simulink model "penduloDobleEnsambleconfunciones"  (R2013a)
settings: Solver=ode45  StartTime=0.0  StopTime=inf  RelTol=1e-3
values from neighbouring files (symbols this model uses):
  g = 9.81    [Parametros_Pendulo_Doble.m]
  Theta1 = (m1*lc1^2)+(m2*l1^2)+I1    (= 0.09775488)    [Parametros_Pendulo_Doble.m]
  Theta2 = (m2*lc2^2)+I2    (= 0.00775807)    [Parametros_Pendulo_Doble.m]
  Theta3 = (m2*l1*lc2)    (= 0.008897)    [Parametros_Pendulo_Doble.m]
  Theta4 = (m1*lc1)+(m2*l1)    (= 0.495148)    [Parametros_Pendulo_Doble.m]
  Theta5 = (m2*lc2)    (= 0.044485)    [Parametros_Pendulo_Doble.m]
undefined symbols (not defined in the file or in its folder): perno
libraries: mblibv1 x16
settings Model: Creator=LornBaltymor  LastModifiedBy=Daniel
settings SimMechanicsCC: VisOnUpdateDiagram=on  VisDuringSimulation=on

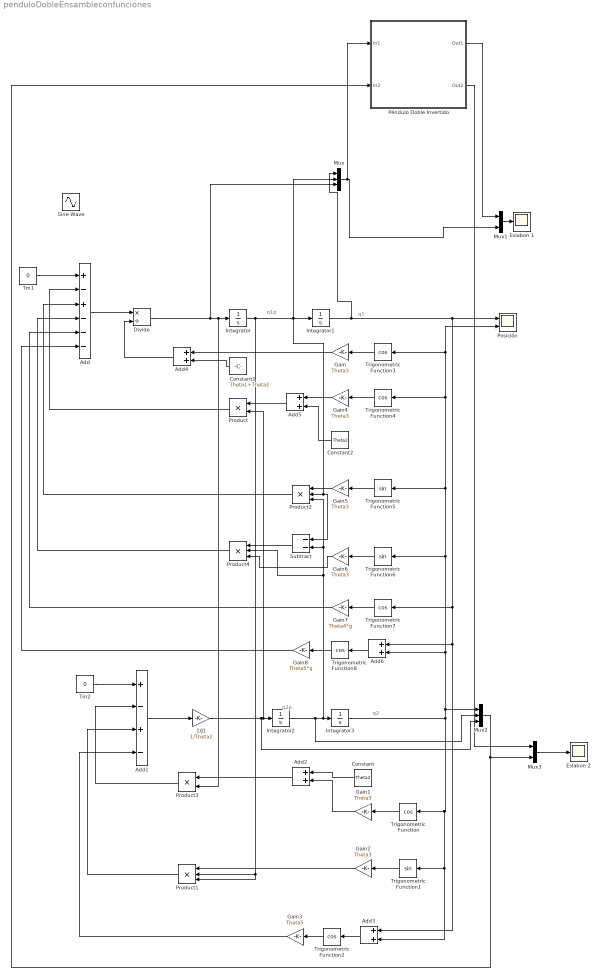
== system penduloDobleEnsambleconfunciones ==
  note: q2
  note: q1
  note: q1p
  note: q2p
  1/J1 : Gain  Gain=1/Theta2
  Add : Sum  Inputs=+-+---
  Add1 : Sum  Inputs=+-+-
  Add{2..6} (5 alike) : Sum
  Constant : Constant  Value=Theta2
  Constant1 : Constant  Value=Theta1+Theta2
  Constant2 : Constant  Value=Theta2
  Divide : Product  Inputs=*/
  Eslabon 1 : Scope
      settings: YMin=-1000  YMax=12000
  "Eslabon 2 " : Scope
      settings: YMin=-1000  YMax=12000  SaveName=ScopeData2
  Gain{,1..2,4..6} (6 alike) : Gain  Gain=Theta3
  Gain3 : Gain  Gain=Theta5
  Gain7 : Gain  Gain=Theta4*g
  Gain8 : Gain  Gain=Theta5*g
  Integrator : Integrator
  Integrator1 : Integrator  InitialCondition=pi/2
  Integrator2 : Integrator
  Integrator3 : Integrator  InitialCondition=pi/2
  Mux : Mux  Inputs=3
  Mux1 : Mux  Inputs=2
  Mux2 : Mux  Inputs=3
  Mux3 : Mux  Inputs=2
  Posición : Scope  NumInputPorts=2
      settings: YMin=86700~-3.21  YMax=88100~-3.07
  Product : Product
  Product1 : Product  Inputs=3
  Product2 : Product  Inputs=3
  Product3 : Product
  Product4 : Product  Inputs=3
  Péndulo Doble Invertido : Subsystem
  Sine Wave : Sin  SampleTime=0
  Subtract : Sum  Inputs=--
  Tm1 : Constant  Value=0
  Tm2 : Constant  Value=0
  Trigonometric Function{,2..4,7..8} (6 alike) : Trigonometry  Operator=cos
  Trigonometric Function1 : Trigonometry
  Trigonometric Function5 : Trigonometry
  Trigonometric Function6 : Trigonometry
  wires:
  Tm2/1 -> Add1/1
  Add1/1 -> 1/J1/1
  1/J1/1 -> Mux2/3, Product/2, Integrator2/1
  Integrator1/1 -> Mux/1, Trigonometric Function7/1, Add6/1, Add3/1, Posición/1
  Integrator2/1 -> Mux2/2, Product4/2, Subtract/2, Product2/3, Integrator3/1
  Divide/1 -> Mux/3, Product3/2, Integrator/1
  Integrator/1 -> Subtract/1, Product2/2, Mux/2, Integrator1/1, Product1/3, Product1/2
  Product3/1 -> Add1/2
  Constant/1 -> Add2/1
  Gain1/1 -> Add2/2
  Trigonometric Function/1 -> Gain1/1
  Integrator3/1 -> Mux2/1, Add6/2, Trigonometric Function6/1, Trigonometric Function5/1, Trigonometric Function4/1, Trigonometric Function3/1, Posición/2, Add3/2, Trigonometric Function1/1, Trigonometric Function/1
  Add2/1 -> Product3/1
  Trigonometric Function1/1 -> Gain2/1
  Gain2/1 -> Product1/1
  Product1/1 -> Add1/3
  Trigonometric Function2/1 -> Gain3/1
  Gain3/1 -> Add1/4
  Add3/1 -> Trigonometric Function2/1
  Trigonometric Function3/1 -> Gain/1
  Gain/1 -> Add4/1
  Constant1/1 -> Add4/2
  Add4/1 -> Divide/2
  Add/1 -> Divide/1
  Trigonometric Function4/1 -> Gain4/1
  Gain4/1 -> Add5/1
  Constant2/1 -> Add5/2
  Add5/1 -> Product/1
  Product/1 -> Add/2
  Trigonometric Function5/1 -> Gain5/1
  Gain5/1 -> Product2/1
  Product2/1 -> Add/3
  Subtract/1 -> Product4/1
  Gain6/1 -> Product4/3
  Trigonometric Function6/1 -> Gain6/1
  Product4/1 -> Add/4
  Trigonometric Function7/1 -> Gain7/1
  Gain7/1 -> Add/5
  Trigonometric Function8/1 -> Gain8/1
  Add6/1 -> Trigonometric Function8/1
  Gain8/1 -> Add/6
  Mux/1 -> Péndulo Doble Invertido/1(In1), Mux1/2
  Mux1/1 -> Eslabon 1/1
  Péndulo Doble Invertido/1(Out1) -> Mux1/1
  Mux2/1 -> Mux3/2, Péndulo Doble Invertido/2(In2)
  Péndulo Doble Invertido/2(Out2) -> Mux3/1
  Mux3/1 -> "Eslabon 2 "/1
  Tm1/1 -> Add/1

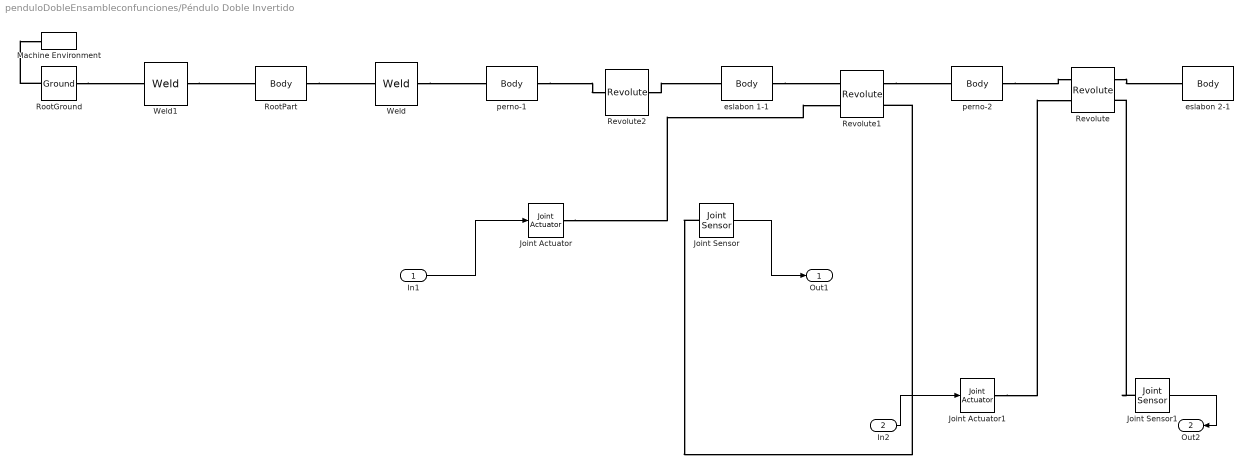
== system penduloDobleEnsambleconfunciones/Péndulo Doble Invertido ==
  In1 : Inport
  In2 : Inport  Port=2
  Joint Actuator : mblibv1/Sensors &  Actuators/Joint Actuator  UpdateFromCAD=off  PhysicalDomain=Mechanical  PortType=blob  ActuationStyle=Motion  AngleUnits=deg  ArcVelocityUnits=deg/s  ArcAccelerationUnits=deg/s^2  CoordPositionUnits=m  VelocityUnits=m/s  AccelerationUnits=m/s^2  ForceUnits=N  TorqueUnits=N*m  ActiveIO=on  Width=3  DialogClass=MechanicalActuatorBlock  Primitive=R1  ReferenceFrame=Absolute (World)
  Joint Actuator1 : mblibv1/Sensors &  Actuators/Joint Actuator  UpdateFromCAD=off  PhysicalDomain=Mechanical  PortType=blob  ActuationStyle=Motion  AngleUnits=deg  ArcVelocityUnits=deg/s  ArcAccelerationUnits=deg/s^2  CoordPositionUnits=m  VelocityUnits=m/s  AccelerationUnits=m/s^2  ForceUnits=N  TorqueUnits=N*m  ActiveIO=on  Width=3  DialogClass=MechanicalActuatorBlock  Primitive=R1  ReferenceFrame=Absolute (World)
  Joint Sensor : mblibv1/Sensors &  Actuators/Joint Sensor  UpdateFromCAD=off  PhysicalDomain=Mechanical  PortType=blob  Muxed=on  Pose=off  Angle=on  AngleUnits=deg  ArcVelocity=off  ArcVelocityUnits=deg/s  ArcAcceleration=off  ArcAccelerationUnits=deg/s^2  CoordPosition=on  CoordPositionUnits=m  Velocity=off  VelocityUnits=m/s  Acceleration=off  AccelerationUnits=m/s^2  Quaternion=on  QuaternionDT=off  QuaternionDDT=off  QuaternionUnits=off  OutputVector=[1]  ActiveIO=on  Width=1  DialogClass=MechanicalSensorBlock  Primitive=R1  Force=off  ForceUnits=N  Torque=off  TorqueUnits=N*m  ReferenceFrame=Absolute (World)  ReactionSensedSide=Base  ReactionReferenceFrame=Absolute (World)  ReactionForce=off  ReactionForceUnits=N  ReactionMoment=off  ReactionMomentUnits=N*m
  Joint Sensor1 : mblibv1/Sensors &  Actuators/Joint Sensor  UpdateFromCAD=off  PhysicalDomain=Mechanical  PortType=blob  Muxed=on  Pose=off  Angle=on  AngleUnits=deg  ArcVelocity=off  ArcVelocityUnits=deg/s  ArcAcceleration=off  ArcAccelerationUnits=deg/s^2  CoordPosition=on  CoordPositionUnits=m  Velocity=off  VelocityUnits=m/s  Acceleration=off  AccelerationUnits=m/s^2  Quaternion=on  QuaternionDT=off  QuaternionDDT=off  QuaternionUnits=off  OutputVector=[1]  ActiveIO=on  Width=1  DialogClass=MechanicalSensorBlock  Primitive=R1  Force=off  ForceUnits=N  Torque=off  TorqueUnits=N*m  ReferenceFrame=Absolute (World)  ReactionSensedSide=Base  ReactionReferenceFrame=Absolute (World)  ReactionForce=off  ReactionForceUnits=N  ReactionMoment=off  ReactionMomentUnits=N*m
  Machine Environment : mblibv1/Bodies/Machine Environment  PortType=env  PhysicalDomain=Mechanical  DialogTemplateClass=MECH.MachineEnvironment  SyncWhenCopied=off  Gravity=[0 -9.81 0]  GravityUnits=m/s^2  GravityAsSignal=off  Dimensionality=Auto-detect  AnalysisType=Forward dynamics  LinearAssemblyTolerance=1e-3  LinearAssemblyToleranceUnits=m  AngularAssemblyTolerance=1e-3  AngularAssemblyToleranceUnits=rad  ConstraintSolverType=Stabilizing  ConstraintRelTolerance=1e-4  ConstraintAbsTolerance=1e-4  UseRobustSingularityHandling=off  RedundancyAnalysisToleranceType=Automatically select tolerance  RedundancyAnalysisTolerance=1e-14  StatePerturbationType=Fixed  PerturbationSize=1e-5  VisualizeMachine=on  BodyVisualizationType=Use model default body geometries  BodyColorSelMode=Use model default  DefaultBodyColor=[1 0 0]
  Revolute : mblibv1/Joints/Revolute  LConnTagsString=__newl0|SA1  RConnTagsString=__newr0|SA1  UpdateFromCAD=on  PMImportedID=eslabon 2-1:-:perno-2  NumSAPorts=2  CutJoint=off  MarkAsCut=off  Primitives=prismatic  PrimitiveProps=R1$World$[0,0,-1]$revolute  DialogClass=JointBlock  R1Axis=[0,0,-1]
  Revolute1 : mblibv1/Joints/Revolute  LConnTagsString=__newl0|SA1  RConnTagsString=__newr0|SA1  UpdateFromCAD=on  PMImportedID=eslabon 1-1:-:perno-2  NumSAPorts=2  CutJoint=off  MarkAsCut=off  Primitives=prismatic  PrimitiveProps=R1$World$[0,0,1]$revolute  DialogClass=JointBlock  R1Axis=[0,0,1]
  Revolute2 : mblibv1/Joints/Revolute  LConnTagsString=__newl0  RConnTagsString=__newr0  UpdateFromCAD=on  PMImportedID=eslabon 1-1:-:perno-1  NumSAPorts=0  CutJoint=off  MarkAsCut=off  Primitives=prismatic  PrimitiveProps=R1$World$[0,0,1]$revolute  DialogClass=JointBlock  R1Axis=[0,0,1]
  RootGround : mblibv1/Bodies/Ground  UpdateFromCAD=on  PMImportedID=RootGround  LeftPortType=env  RightPortType=workingframe  PhysicalDomain=Mechanical  DialogClass=GroundBlock  CoordPosition=[0.0411534,0.0510219,0.0512834]  CoordPositionUnits=m  StateVectorMgrId=2  MachineId=[3 0]  ShowEnvPort=on
  RootPart : mblibv1/Bodies/Body  LConnTagsString=CS3  RConnTagsString=CS2  UpdateFromCAD=on  PMImportedID=pendulo doble ensamble/RootPart  DialogClass=MechanicalBodyBlock  Mass=0  MassUnits=kg  InertiaUnits=kg*m^2  Inertia=[0,0,0;0,0,0;0,0,0]  Shape=Cylinder  ShapeDims=[1 1]  ShapeUnits=m  ShapeUse=false  Density=1  DensityUnits=kg/m^3  DensityUse=false  GraphicsMode=MACHINE_DEFAULT  BodyColorSelMode=MACHINE_DEFAULT  BodyColor=[1;0;0]  AttachedToCS=CS1  CG=Right$CG$[0.0411534 0.0510219 0.0512834]$WORLD$WORLD$m$[1 0 0;0 1 0;0 0 1]$3x3 Transform$rad$WORLD$false$pendulo doble ensamble/RootPart::CG(AUTOGEN)  WorkingFrames=Right$CS1$[0 0 0]$WORLD$WORLD$m$[1 0 0;0 1 0;0 0 1]$3x3 Transform$rad$WORLD$false$pendulo doble ensamble/RootPart::CS1(AUTOGEN)#Right$CS2$[0.000634377 -0.00147675 0.05]$WORLD$WORLD$m$[1 0 0;0 1 0;0 0 1]$3x3 Transform$rad$WORLD$true$pendulo doble ensamble/RootPart:-:perno-1::pendulo doble ensamble/RootPart(AUTOGEN)#Left$CS3$[0.0411534 0.0510219 0.0512834]$WORLD$WORLD$m$[1 0 0;0 1 0;0 0 1]$3x3 Transform$rad$WORLD$true$RootGround:-:pendulo doble ensamble/RootPart::pendulo doble ensamble/RootPart(AUTOGEN)  CGPos=[0.0411534 0.0510219 0.0512834]  CGRot=[1 0 0;0 1 0;0 0 1]  CS0Pos=[]  CS0Rot=[]  CS1Pos=[0 0 0]  CS1Rot=[1 0 0;0 1 0;0 0 1]  CS2Pos=[0.000634377 -0.00147675 0.05]  CS2Rot=[1 0 0;0 1 0;0 0 1]  CS3Pos=[0.0411534 0.0510219 0.0512834]  CS3Rot=[1 0 0;0 1 0;0 0 1]  CS4Pos=[]  CS4Rot=[]  CS5Pos=[]  CS5Rot=[]  CS6Pos=[]  CS6Rot=[]  CS7Pos=[]  CS7Rot=[]  CS8Pos=[]  CS8Rot=[]  CS9Pos=[]  CS9Rot=[]  CS10Pos=[]  CS10Rot=[]  CS11Pos=[]  CS11Rot=[]  CS12Pos=[]  CS12Rot=[]  CS13Pos=[]  CS13Rot=[]  CS14Pos=[]  CS14Rot=[]  CS15Pos=[]  CS15Rot=[]  CS16Pos=[]  CS16Rot=[]  CS17Pos=[]  CS17Rot=[]  CS18Pos=[]  CS18Rot=[]  CS19Pos=[]  CS19Rot=[]  CS20Pos=[]  CS20Rot=[]
  Weld : mblibv1/Joints/Weld  LConnTagsString=__newl0  RConnTagsString=__newr0  UpdateFromCAD=on  PMImportedID=pendulo doble ensamble/RootPart:-:perno-1  NumSAPorts=0  CutJoint=off  MarkAsCut=off  Primitives=weld  PrimitiveProps=W$WORLD$[0.57735,0.57735,0.57735]$weld  DialogClass=JointBlock  WAxis=[0.57735,0.57735,0.57735]
  Weld1 : mblibv1/Joints/Weld  LConnTagsString=__newl0  RConnTagsString=__newr0  UpdateFromCAD=on  PMImportedID=RootGround:-:pendulo doble ensamble/RootPart  NumSAPorts=0  CutJoint=off  MarkAsCut=off  Primitives=weld  PrimitiveProps=W$WORLD$[0.57735,0.57735,0.57735]$weld  DialogClass=JointBlock  WAxis=[0.57735,0.57735,0.57735]
  eslabon 1-1 : mblibv1/Bodies/Body  LConnTagsString=CS3  RConnTagsString=CS2  UpdateFromCAD=on  PMImportedID=eslabon 1-1  DialogClass=MechanicalBodyBlock  Mass=0.0368584  MassUnits=kg  InertiaUnits=kg*m^2  Inertia=[2.95158e-05,0,0;0,2.54231e-06,0;0,0,2.96008e-05]  Shape=Cylinder  ShapeDims=[1 1]  ShapeUnits=m  ShapeUse=false  Density=1  DensityUnits=kg/m^3  DensityUse=false  GraphicsMode=GFXFILE  GraphicsFileName=pendulo doble ensamble - eslabon 1-1.STL  BodyColorSelMode=COLORPALETTE  BodyColor=[0.792157;0.819608;0.933333]  AttachedToCS=CS1  CG=Right$CG$[0.0289122 0.0268139 0.065]$WORLD$WORLD$m$[-0.707267 -0.706946 0;0.706946 -0.707267 0;0 0 1]$3x3 Transform$rad$WORLD$false$eslabon 1-1::CG(AUTOGEN)  WorkingFrames=Right$CS1$[0.0642596 0.0621773 0.065]$WORLD$WORLD$m$[-0.707267 -0.706946 0;0.706946 -0.707267 0;0 0 1]$3x3 Transform$rad$WORLD$false$eslabon 1-1::CS1(AUTOGEN)#Right$CS2$[0.0571901 0.0551046 0.075]$WORLD$WORLD$m$[1 0 0;0 1 0;0 0 1]$3x3 Transform$rad$WORLD$true$eslabon 1-1:-:perno-2::eslabon 1-1(AUTOGEN)#Left$CS3$[0.000634377 -0.00147675 0.075]$WORLD$WORLD$m$[1 0 0;0 1 0;0 0 1]$3x3 Transform$rad$WORLD$true$eslabon 1-1:-:perno-1::eslabon 1-1(AUTOGEN)  CGPos=[0.0289122 0.0268139 0.065]  CGRot=[-0.707267 -0.706946 0;0.706946 -0.707267 0;0 0 1]  CS0Pos=[]  CS0Rot=[]  CS1Pos=[0.0642596 0.0621773 0.065]  CS1Rot=[-0.707267 -0.706946 0;0.706946 -0.707267 0;0 0 1]  CS2Pos=[0.0571901 0.0551046 0.075]  CS2Rot=[1 0 0;0 1 0;0 0 1]  CS3Pos=[0.000634377 -0.00147675 0.075]  CS3Rot=[1 0 0;0 1 0;0 0 1]  CS4Pos=[]  CS4Rot=[]  CS5Pos=[]  CS5Rot=[]  CS6Pos=[]  CS6Rot=[]  CS7Pos=[]  CS7Rot=[]  CS8Pos=[]  CS8Rot=[]  CS9Pos=[]  CS9Rot=[]  CS10Pos=[]  CS10Rot=[]  CS11Pos=[]  CS11Rot=[]  CS12Pos=[]  CS12Rot=[]  CS13Pos=[]  CS13Rot=[]  CS14Pos=[]  CS14Rot=[]  CS15Pos=[]  CS15Rot=[]  CS16Pos=[]  CS16Rot=[]  CS17Pos=[]  CS17Rot=[]  CS18Pos=[]  CS18Rot=[]  CS19Pos=[]  CS19Rot=[]  CS20Pos=[]  CS20Rot=[]
  eslabon 2-1 : mblibv1/Bodies/Body  LConnTagsString=CS2  UpdateFromCAD=on  PMImportedID=eslabon 2-1  DialogClass=MechanicalBodyBlock  Mass=0.0304292  MassUnits=kg  InertiaUnits=kg*m^2  Inertia=[1.65845e-05,0,0;0,2.07116e-06,0;0,0,1.6627e-05]  Shape=Cylinder  ShapeDims=[1 1]  ShapeUnits=m  ShapeUse=false  Density=1  DensityUnits=kg/m^3  DensityUse=false  GraphicsMode=GFXFILE  GraphicsFileName=pendulo doble ensamble - eslabon 2-1.STL  BodyColorSelMode=COLORPALETTE  BodyColor=[0.792157;0.819608;0.933333]  AttachedToCS=CS1  CG=Right$CG$[0.0591404 0.0865929 0.035]$WORLD$WORLD$m$[-0.998087 -0.0618188 0;0.0618188 -0.998087 0;0 0 1]$3x3 Transform$rad$WORLD$false$eslabon 2-1::CG(AUTOGEN)  WorkingFrames=Right$CS1$[0.0615174 0.124971 0.035]$WORLD$WORLD$m$[-0.998087 -0.0618188 0;0.0618188 -0.998087 0;0 0 1]$3x3 Transform$rad$WORLD$false$eslabon 2-1::CS1(AUTOGEN)#Left$CS2$[0.0571901 0.0551046 0.025]$WORLD$WORLD$m$[1 0 0;0 1 0;0 0 1]$3x3 Transform$rad$WORLD$true$eslabon 2-1:-:perno-2::eslabon 2-1(AUTOGEN)  CGPos=[0.0591404 0.0865929 0.035]  CGRot=[-0.998087 -0.0618188 0;0.0618188 -0.998087 0;0 0 1]  CS0Pos=[]  CS0Rot=[]  CS1Pos=[0.0615174 0.124971 0.035]  CS1Rot=[-0.998087 -0.0618188 0;0.0618188 -0.998087 0;0 0 1]  CS2Pos=[0.0571901 0.0551046 0.025]  CS2Rot=[1 0 0;0 1 0;0 0 1]  CS3Pos=[]  CS3Rot=[]  CS4Pos=[]  CS4Rot=[]  CS5Pos=[]  CS5Rot=[]  CS6Pos=[]  CS6Rot=[]  CS7Pos=[]  CS7Rot=[]  CS8Pos=[]  CS8Rot=[]  CS9Pos=[]  CS9Rot=[]  CS10Pos=[]  CS10Rot=[]  CS11Pos=[]  CS11Rot=[]  CS12Pos=[]  CS12Rot=[]  CS13Pos=[]  CS13Rot=[]  CS14Pos=[]  CS14Rot=[]  CS15Pos=[]  CS15Rot=[]  CS16Pos=[]  CS16Rot=[]  CS17Pos=[]  CS17Rot=[]  CS18Pos=[]  CS18Rot=[]  CS19Pos=[]  CS19Rot=[]  CS20Pos=[]  CS20Rot=[]
  perno-1 : mblibv1/Bodies/Body  LConnTagsString=CS2  RConnTagsString=CS3  UpdateFromCAD=on  PMImportedID=perno-1  DialogClass=MechanicalBodyBlock  Mass=0.00392699  MassUnits=kg  InertiaUnits=kg*m^2  Inertia=[8.42667e-07,0,0;0,8.42667e-07,0;0,0,4.90874e-08]  Shape=Cylinder  ShapeDims=[1 1]  ShapeUnits=m  ShapeUse=false  Density=1  DensityUnits=kg/m^3  DensityUse=false  GraphicsMode=GFXFILE  GraphicsFileName=pendulo doble ensamble - perno-1.STL  BodyColorSelMode=COLORPALETTE  BodyColor=[0.792157;0.819608;0.933333]  AttachedToCS=CS1  CG=Right$CG$[0.000634377 -0.00147675 0.05]$WORLD$WORLD$m$[1 0 0;0 1 0;0 0 1]$3x3 Transform$rad$WORLD$false$perno-1::CG(AUTOGEN)  WorkingFrames=Right$CS1$[0.000634377 -0.00147675 0.075]$WORLD$WORLD$m$[1 0 0;0 1 0;0 0 1]$3x3 Transform$rad$WORLD$false$perno-1::CS1(AUTOGEN)#Left$CS2$[0.000634377 -0.00147675 0.05]$WORLD$WORLD$m$[1 0 0;0 1 0;0 0 1]$3x3 Transform$rad$WORLD$true$pendulo doble ensamble/RootPart:-:perno-1::perno-1(AUTOGEN)#Right$CS3$[0.000634377 -0.00147675 0.075]$WORLD$WORLD$m$[1 0 0;0 1 0;0 0 1]$3x3 Transform$rad$WORLD$true$eslabon 1-1:-:perno-1::perno-1(AUTOGEN)  CGPos=[0.000634377 -0.00147675 0.05]  CGRot=[1 0 0;0 1 0;0 0 1]  CS0Pos=[]  CS0Rot=[]  CS1Pos=[0.000634377 -0.00147675 0.075]  CS1Rot=[1 0 0;0 1 0;0 0 1]  CS2Pos=[0.000634377 -0.00147675 0.05]  CS2Rot=[1 0 0;0 1 0;0 0 1]  CS3Pos=[0.000634377 -0.00147675 0.075]  CS3Rot=[1 0 0;0 1 0;0 0 1]  CS4Pos=[]  CS4Rot=[]  CS5Pos=[]  CS5Rot=[]  CS6Pos=[]  CS6Rot=[]  CS7Pos=[]  CS7Rot=[]  CS8Pos=[]  CS8Rot=[]  CS9Pos=[]  CS9Rot=[]  CS10Pos=[]  CS10Rot=[]  CS11Pos=[]  CS11Rot=[]  CS12Pos=[]  CS12Rot=[]  CS13Pos=[]  CS13Rot=[]  CS14Pos=[]  CS14Rot=[]  CS15Pos=[]  CS15Rot=[]  CS16Pos=[]  CS16Rot=[]  CS17Pos=[]  CS17Rot=[]  CS18Pos=[]  CS18Rot=[]  CS19Pos=[]  CS19Rot=[]  CS20Pos=[]  CS20Rot=[]
  perno-2 : mblibv1/Bodies/Body  LConnTagsString=CS3  RConnTagsString=CS2  UpdateFromCAD=on  PMImportedID=perno-2  DialogClass=MechanicalBodyBlock  Mass=0.00392699  MassUnits=kg  InertiaUnits=kg*m^2  Inertia=[8.42667e-07,0,0;0,8.42667e-07,0;0,0,4.90874e-08]  Shape=Cylinder  ShapeDims=[1 1]  ShapeUnits=m  ShapeUse=false  Density=1  DensityUnits=kg/m^3  DensityUse=false  GraphicsMode=GFXFILE  GraphicsFileName=pendulo doble ensamble - perno-2.STL  BodyColorSelMode=COLORPALETTE  BodyColor=[0.792157;0.819608;0.933333]  AttachedToCS=CS1  CG=Right$CG$[0.0571901 0.0551046 0.05]$WORLD$WORLD$m$[-0.760616 0.649202 0;-0.649202 -0.760616 0;0 0 1]$3x3 Transform$rad$WORLD$false$perno-2::CG(AUTOGEN)  WorkingFrames=Right$CS1$[0.0571901 0.0551046 0.075]$WORLD$WORLD$m$[-0.760616 0.649202 0;-0.649202 -0.760616 0;0 0 1]$3x3 Transform$rad$WORLD$false$perno-2::CS1(AUTOGEN)#Right$CS2$[0.0571901 0.0551046 0.025]$WORLD$WORLD$m$[1 0 0;0 1 0;0 0 1]$3x3 Transform$rad$WORLD$true$eslabon 2-1:-:perno-2::perno-2(AUTOGEN)#Left$CS3$[0.0571901 0.0551046 0.075]$WORLD$WORLD$m$[1 0 0;0 1 0;0 0 1]$3x3 Transform$rad$WORLD$true$eslabon 1-1:-:perno-2::perno-2(AUTOGEN)  CGPos=[0.0571901 0.0551046 0.05]  CGRot=[-0.760616 0.649202 0;-0.649202 -0.760616 0;0 0 1]  CS0Pos=[]  CS0Rot=[]  CS1Pos=[0.0571901 0.0551046 0.075]  CS1Rot=[-0.760616 0.649202 0;-0.649202 -0.760616 0;0 0 1]  CS2Pos=[0.0571901 0.0551046 0.025]  CS2Rot=[1 0 0;0 1 0;0 0 1]  CS3Pos=[0.0571901 0.0551046 0.075]  CS3Rot=[1 0 0;0 1 0;0 0 1]  CS4Pos=[]  CS4Rot=[]  CS5Pos=[]  CS5Rot=[]  CS6Pos=[]  CS6Rot=[]  CS7Pos=[]  CS7Rot=[]  CS8Pos=[]  CS8Rot=[]  CS9Pos=[]  CS9Rot=[]  CS10Pos=[]  CS10Rot=[]  CS11Pos=[]  CS11Rot=[]  CS12Pos=[]  CS12Rot=[]  CS13Pos=[]  CS13Rot=[]  CS14Pos=[]  CS14Rot=[]  CS15Pos=[]  CS15Rot=[]  CS16Pos=[]  CS16Rot=[]  CS17Pos=[]  CS17Rot=[]  CS18Pos=[]  CS18Rot=[]  CS19Pos=[]  CS19Rot=[]  CS20Pos=[]  CS20Rot=[]
  Out1 : Outport
  Out2 : Outport  Port=2
  wires:
  In1/1 -> Joint Actuator/1
  Joint Sensor/1 -> Out1/1
  In2/1 -> Joint Actuator1/1
  Joint Sensor1/1 -> Out2/1
  connections:
  Revolute/RConn1 -- eslabon 2-1/LConn1
  Revolute2/RConn1 -- eslabon 1-1/LConn1
  RootPart/RConn1 -- Weld/LConn1
  Weld/RConn1 -- perno-1/LConn1
  Weld1/RConn1 -- RootPart/LConn1
  perno-2/RConn1 -- Revolute/LConn1
  perno-1/RConn1 -- Revolute2/LConn1
  Revolute1/RConn1 -- perno-2/LConn1
  RootGround/RConn1 -- Weld1/LConn1
  eslabon 1-1/RConn1 -- Revolute1/LConn1
  RootGround/LConn1 -- Machine Environment/RConn1
  Joint Actuator/RConn1 -- Revolute1/LConn2
  Joint Sensor/LConn1 -- Revolute1/RConn2
  Joint Actuator1/RConn1 -- Revolute/LConn2
  Joint Sensor1/LConn1 -- Revolute/RConn2
